simulink model "Ex2"  (R2024b)
settings: Solver=VariableStepAuto  StartTime=0.0  StopTime=10.0  RelTol=1e-3
values from neighbouring files (symbols this model uses):
  A = [0 1 0 0 0 0;-(K1+K2+K3)/M1 -(C1+C2+C3)/M1 K2/M1 C2/M1 K3/M1 C3/M1;     0 0 0 1 0 0; K2/M2 C2/M2 -(K2+K4+K5)/M2 -(C2+C4+C5)/M2 K4/M2 C4/M2;     0 0 0 0 0 1;K5/M3 C3/M3 K4/M3 C4/M3 -(K3+K4)/M3 -(C3+C4)/M3]    [Tp1.m]
  B = [0; 0; 0 ; 1/M2; 0; 0 ]    [Tp1.m]
  C = [eye(6)]    [Tp1.m]
  D = [0;0;0;0;0;0]    [Tp1.m]
  K = place(A,B,P)    [Tp1.m]
  x0 = [x10;0;x20;0;x30;0]    [Tp1.m]
libraries: fl_lib x18, nesl_utility x5
settings Model: Creator=magne
settings RTWCC: GPUComputeCapability=3.5

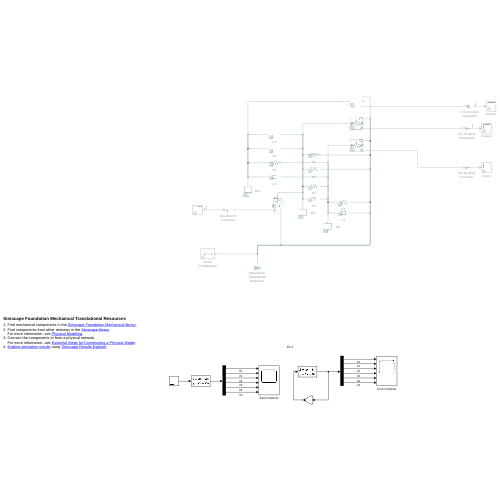
[thumbnail: Simulink's stored preview of the top-level diagram]
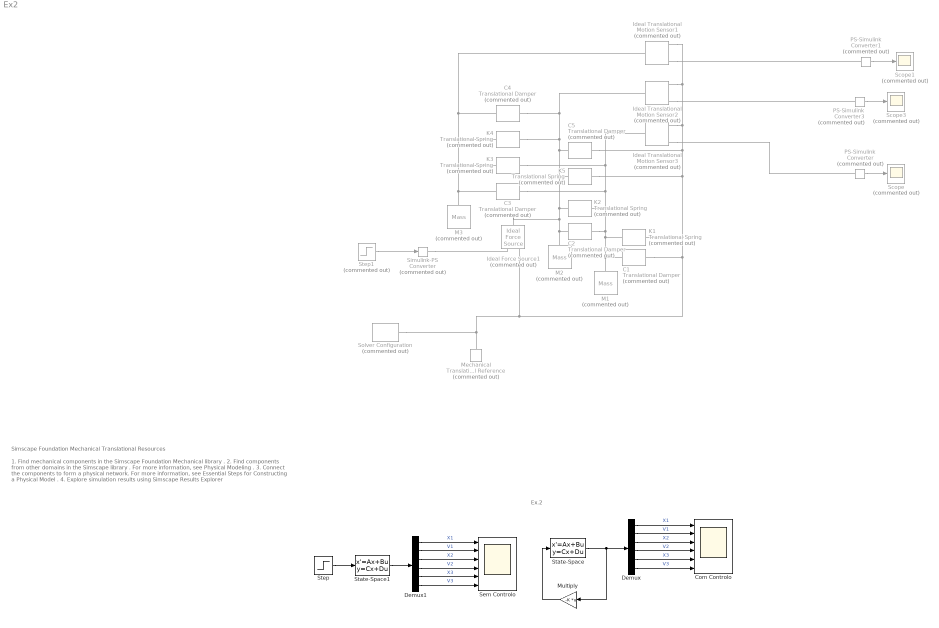
== system Ex2 ==
  note: Ex.2
  note: 1. Find mechanical components in the Simscape Foundation Mechanical library .
      | 2. Find components from other domains in the Simscape library .
      | For more information, see Physical Modeling .
      | 3. Connect the components to form a physical network.
      | For more information, see Essential Steps for Constructing a Physical Model .
      | 4. Explore simulation results using Simscape Results Explorer
  note: Simscape Foundation Mechanical Translational Resources
  C{1..5} (5 alike) : fl_lib/Mechanical/Translational Elements/Translational Damper  Commented=on  D=100 N*s/m  v_specify=off  v_priority=None  v=0 m/s  v_nominal_specify=off  v_nominal_value=1  v_nominal_unit=m/s  f_specify=off  f_priority=None  f=0 N  f_nominal_specify=off  f_nominal_value=1  f_nominal_unit=N
  Com Controlo : Scope  NumInputPorts=6
  Demux : Demux  Outputs=6
  Demux1 : Demux  Outputs=6
  Ideal Force Source1 : fl_lib/Mechanical/Mechanical Sources/Ideal Force Source  Commented=on
  Ideal Translational Motion Sensor1 : fl_lib/Mechanical/Mechanical Sensors/Ideal Translational Motion Sensor  Commented=on  reference=foundation.enum.MeasurementReference.difference  acceleration_port=false  velocity_port=true  position_port=true  offset=0 m
  Ideal Translational Motion Sensor2 : fl_lib/Mechanical/Mechanical Sensors/Ideal Translational Motion Sensor  Commented=on  reference=foundation.enum.MeasurementReference.difference  acceleration_port=false  velocity_port=true  position_port=true  offset=0 m
  Ideal Translational Motion Sensor3 : fl_lib/Mechanical/Mechanical Sensors/Ideal Translational Motion Sensor  Commented=on  reference=foundation.enum.MeasurementReference.difference  acceleration_port=false  velocity_port=true  position_port=true  offset=0 m
  K{1..5} (5 alike) : fl_lib/Mechanical/Translational Elements/Translational Spring  Commented=on  spr_rate=1000 N/m  v_specify=off  v_priority=None  v=0 m/s  v_nominal_specify=off  v_nominal_value=1  v_nominal_unit=m/s  f_specify=off  f_priority=None  f=0 N  f_nominal_specify=off  f_nominal_value=1  f_nominal_unit=N  x_specify=off  x_priority=High  x=0 m  x_nominal_specify=off  x_nominal_value=1  x_nominal_unit=m
  M1 : fl_lib/Mechanical/Translational Elements/Mass  Commented=on  mass=1 kg  num_ports=foundation.enum.numPorts2.one  v_specify=off  v_priority=High  v=0 m/s  v_nominal_specify=off  v_nominal_value=1  v_nominal_unit=m/s  f_specify=off  f_priority=None  f=0 N  f_nominal_specify=off  f_nominal_value=1  f_nominal_unit=N
  M2 : fl_lib/Mechanical/Translational Elements/Mass  Commented=on  mass=1 kg  num_ports=foundation.enum.numPorts2.one  v_specify=off  v_priority=High  v=0 m/s  v_nominal_specify=off  v_nominal_value=1  v_nominal_unit=m/s  f_specify=off  f_priority=None  f=0 N  f_nominal_specify=off  f_nominal_value=1  f_nominal_unit=N
  M3 : fl_lib/Mechanical/Translational Elements/Mass  Commented=on  mass=1 kg  num_ports=foundation.enum.numPorts2.one  v_specify=off  v_priority=High  v=0 m/s  v_nominal_specify=off  v_nominal_value=1  v_nominal_unit=m/s  f_specify=off  f_priority=None  f=0 N  f_nominal_specify=off  f_nominal_value=1  f_nominal_unit=N
  Mechanical Translational Reference : fl_lib/Mechanical/Translational Elements/Mechanical Translational Reference  Commented=on
  Multiply : Gain  Gain=-K  Multiplication=Matrix(K*u) (u vector)
  PS-Simulink Converter : nesl_utility/PS-Simulink Converter  Commented=on  PhysicalDomain=network_engine_domain  SubClassName=ps_output  LeftPortType=input  RightPortType=output  PseudoPeriodic=off  Frequencies=[]  VectorFormat=inherit  Unit=inherit  AffineConversion=off
  PS-Simulink Converter1 : nesl_utility/PS-Simulink Converter  Commented=on  PhysicalDomain=network_engine_domain  SubClassName=ps_output  LeftPortType=input  RightPortType=output  PseudoPeriodic=off  Frequencies=[]  VectorFormat=inherit  Unit=inherit  AffineConversion=off
  PS-Simulink Converter3 : nesl_utility/PS-Simulink Converter  Commented=on  PhysicalDomain=network_engine_domain  SubClassName=ps_output  LeftPortType=input  RightPortType=output  PseudoPeriodic=off  Frequencies=[]  VectorFormat=inherit  Unit=inherit  AffineConversion=off
  Scope : Scope  Commented=on
  Scope1 : Scope  Commented=on
  Scope3 : Scope  Commented=on
  Sem Controlo : Scope  NumInputPorts=6
  Simulink-PS Converter : nesl_utility/Simulink-PS Converter  Commented=on  PhysicalDomain=network_engine_domain  SubClassName=ps_input  LeftPortType=input  RightPortType=output  PseudoPeriodic=off  Frequencies=[]  NoiseDistribution=none  NoiseParameters=[]  Unit=1  AffineConversion=off  FilteringAndDerivatives=provide  SimscapeFilterOrder=1  InputFilterTimeConstant=0.001  UdotUserProvided=0
  Solver Configuration : nesl_utility/Solver Configuration  Commented=on  PhysicalDomain=network_engine_domain  SubClassName=solver  LeftPortType=input  RightPortType=generic  Tones=[]  Harmonics=[]  SimulateNoise=off  Profile=off  UseLocalSampling=off  EnableSwitchedLinearOptims=on  FrequencyDomain=off  UseCCode=off  RelTol=0.001  AbsTol=1e-06  MinStep=1e-09  ToWorkspace=off  RevertToSquareIcSolve=off  NumHomotopyIterations=100  PhasorMode=off  PhasorModeNumHarmonics=1  ConsistencySolver=NEWTON_XTOL_AFTER_FTOL  IndexReductionMethod=DerivativeReplacement  DoDC=off  ResidualTolerance=1e-09  ConsistencyTolSource=GLOBAL  ConsistencyAbsTol=0.001  ConsistencyRelTol=0.001  ConsistencyTolFactor=0.001  UseLocalSolver=off  LocalSolverChoice=NE_BACKWARD_EULER_ADVANCER  ResolveIndetEquations=on  FunctionEvalNumThread=1  LocalSolverSampleTime=0.001  DoFixedCost=off  MaxNonlinIter=3  MaxModeIter=2  ComputeImpulses=off  ImpulseIterations=2  LinearAlgebra=auto  LinearAlgebraNumThread=0  EquationFormulation=NE_TIME_EF  DelaysMemoryBudget=1024  AutomaticFiltering=on  FilteringTimeConstant=0.001  PartitionStorageMethod=AS_NEEDED  PartitionMemoryBudget=1024  PartitionMethod=ROBUST  MultibodyUseLocalSolver=off  MultibodyLocalSolverChoice=ODE1  MultibodyLocalSolverSampleTime=0.001
  State-Space : StateSpace  A=A  B=B  C=C  D=D  InitialCondition=x0
  State-Space1 : StateSpace  A=A  B=B  C=C  D=D  InitialCondition=x0
  Step : Step  SampleTime=0
  Step1 : Step  Commented=on  SampleTime=0
  wires:
  PS-Simulink Converter1/1 -> Scope1/1
  PS-Simulink Converter/1 -> Scope/1
  PS-Simulink Converter3/1 -> Scope3/1
  Step1/1 -> Simulink-PS Converter/1
  Multiply/1 -> State-Space/1
  State-Space/1 -> Multiply/1, Demux/1
  Demux/1 -> Com Controlo/1  "X1"
  Demux/2 -> Com Controlo/2  "V1"
  Demux/3 -> Com Controlo/3  "X2"
  Demux/4 -> Com Controlo/4  "V2"
  Demux/6 -> Com Controlo/6  "V3"
  Demux/5 -> Com Controlo/5  "X3"
  Demux1/5 -> Sem Controlo/5  "X3"
  Demux1/6 -> Sem Controlo/6  "V3"
  Demux1/4 -> Sem Controlo/4  "V2"
  Demux1/3 -> Sem Controlo/3  "X2"
  Demux1/2 -> Sem Controlo/2  "V1"
  Demux1/1 -> Sem Controlo/1  "X1"
  State-Space1/1 -> Demux1/1
  Step/1 -> State-Space1/1
  connections:
  K2/RConn1 -- K3/RConn1 -- Ideal Translational Motion Sensor3/LConn1 -- C3/RConn1 -- C2/RConn1 -- M1/LConn1 -- C1/LConn1 -- K1/LConn1
  K1/RConn1 -- C5/RConn1 -- Ideal Translational Motion Sensor3/RConn1 -- Ideal Translational Motion Sensor1/RConn1 -- Ideal Translational Motion Sensor2/RConn1 -- K5/RConn1 -- C1/RConn1 -- Ideal Force Source1/RConn2 -- Solver Configuration/RConn1 -- Mechanical Translational Reference/LConn1
  K2/LConn1 -- C4/RConn1 -- Ideal Translational Motion Sensor2/LConn1 -- K4/RConn1 -- C5/LConn1 -- K5/LConn1 -- Ideal Force Source1/LConn1 -- C2/LConn1 -- M2/LConn1
  K3/LConn1 -- M3/LConn1 -- C3/LConn1 -- C4/LConn1 -- Ideal Translational Motion Sensor1/LConn1 -- K4/LConn1
  Ideal Translational Motion Sensor3/RConn3 -- PS-Simulink Converter/LConn1
  Ideal Translational Motion Sensor2/RConn3 -- PS-Simulink Converter3/LConn1
  Ideal Translational Motion Sensor1/RConn3 -- PS-Simulink Converter1/LConn1
  Simulink-PS Converter/RConn1 -- Ideal Force Source1/RConn1
